simulink library "MidrangeBtc"  (R2022b)
settings: Solver=VariableStepAuto  StartTime=0.0  StopTime=10.0  RelTol=1e-3
undefined symbols (not defined in the file or in its folder): Row
libraries: TuneVar x14, TOP x4, HandyTextFile x2, SetDsm x2, AudioStats x1, FeaturePath x1, RTC x1
settings Model: Creator=st51187  LastModifiedBy=kl13806
settings SolverCC: AlgebraicLoopSolver=TrustRegion
settings DebuggingCC: UnconnectedInputMsg=warning  UnconnectedOutputMsg=warning  UnconnectedLineMsg=warning  SFMachineParentedDataDiag=warning
settings ModelReferenceCC: EnableRefExpFcnMdlSchedulingChecks=on
settings RTWCC: DLArmComputeVersion=19.05

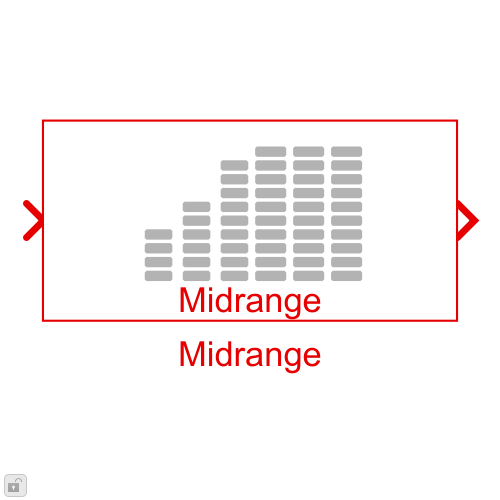
[thumbnail: Simulink's stored preview of the top-level diagram]
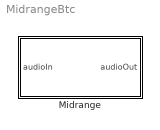
== system MidrangeBtc ==
  Midrange : Subsystem  mask(Blocklib Midrange){FeatureName=Midrange, Config=[]}
      mask prompts: FeatureName "Feature path name:"; Config "MidrangeConfig"
      mask help: The midrange block performs tone controls across midrange frequencies across multiple channels via a 2nd order IIR filter.
      mask init:
      | blkh=gcbh;
      | Config=BTConfig.Assert(blkh,Config);
      | MaskBlockHandle = gcbh;
      | 
      | MidrangeMask.Init(blkh);
      | 
      | % Set boundary conditions
      | rampRateBounds = [5,50000];
      | rampTimeBounds = [1,3000];
      | 
      | BTConfig.InitSetFeatureIfPresent(blkh,'FeatureName');
      | Config.Validate();
      mask Help:
      | The midrange block performs tone controls across midrange frequencies across multiple channels via a 2nd order IIR filter. The midrange content can either be 'boosted' or 'cut' depending on the value of the gain. Different filters can be used for the boost and cut regions, each with its own center frequency and Q value.
      | 
      | MASK PARAMETERS:
      | - Different filter coefficients can be applied for the boost and cut regions (typical center frequency - 775 Hz, Q - 0.9)
      | - The maximum boost/ cut can be specified (typically 20 dB and -20 dB)
      | - The offset and scale values determine the piecewise linear curve that is used to compute the gain (typically 128 and 127 respectively)
      | 
      | RTC CONTROL:
      | Run time control is available to dynamically change the gain to be applied to the midrange content. An index (typically between 0-255) can be provided along with a ramp time and rate (rate gets precedence).
      | RTC_SIM_OBJ.AddREQ( 'MidrangeSet', 0.6, [0005,  <midrange_index>, <ramp_db_per_second>, <ramp_time>]);
      | E.g., RTC_SIM_OBJ.AddREQ( 'MidrangeSet', 0.6, [0005,  50, 0, 50]);
      mask TypeOptions FeatureName: FeaturePath/FeatureName
      mask Callback Config: BTConfig.CallbackHideIfPresent(gcbh,{'FeatureName'});
      mask Display:
      | [path w h] = IconToneMask();
      | 
      | % retrieve the block's pixel size
      | pos = get(gcbh,'position');
      | bw = pos(3) - pos(1);
      | bh = pos(4) - pos(2);
      | 
      | % draw centered icon
      | xAdj = bw/2 - w/2;
      | yAdj = bh/2 - h/2 + 4;
      | for i=1:length(path)
      | 	patch(path(i).x+xAdj, path(i).y+yAdj, path(i).rgb);
      | end
      | 
      | % place feature name text
      | 	text(bw*0.5, 0, ['\n' FeatureName '\n\n'], 'horizontalAlignment', 'center');

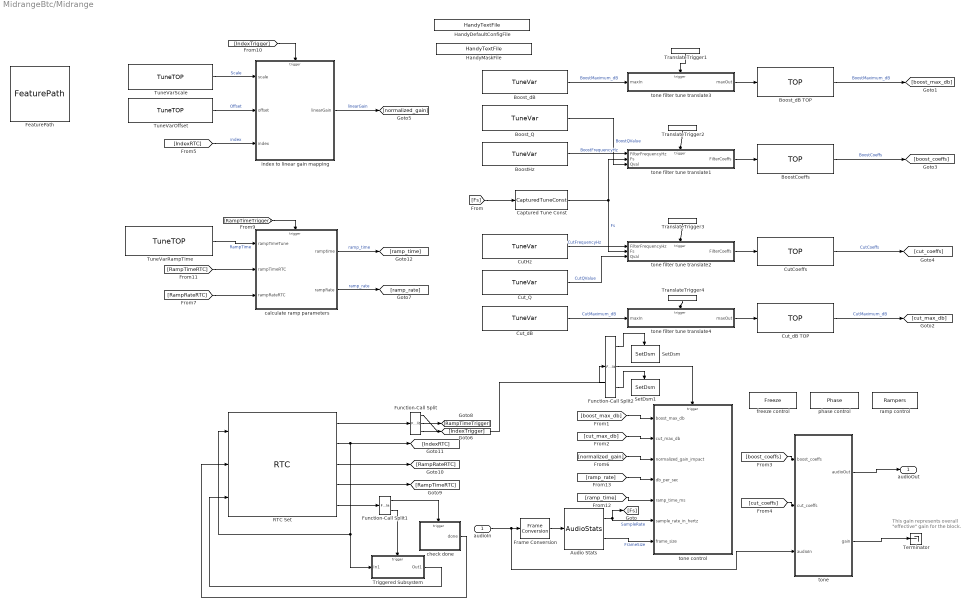
== system MidrangeBtc/Midrange ==
  note: This gain represents overall
      | "effective" gain for the block.
  audioIn : Inport
  Audio Stats : AudioStats/AudioStats  DoSampleRate=on  TypeSampleRate=Inherit: auto  DoCallRate=off  TypeCallRate=Inherit: auto  DoFrameSize=on  TypeFrameSize=Inherit: auto  DoChannelCount=off  TypeChannelCount=Inherit: auto  DoTaskRateFactor=off  TypeTaskRateFactor=Inherit: auto  MacroNameRoot=AUDIO  MacroNameRootEval='AUDIO'  IsMacroNameEval=off  MacroSampleRate=off  MacroCallRate=off  MacroFrameSize=off  MacroChannelCount=off  MacroTaskRateFactor=off  MacroTaskId=off  ValidateSampleRate=off  ValueSampleRate=44100  ValidateCallRate=off  ValueCallRate=[]  ValidateFrameSize=off  ValueFrameSize=32  ValidateChannelCount=off  ValueChannelCount=[]  ValidateTaskRateFactor=off  ValueTaskRateFactor=[]
      settings: SourceProductName=Bose Talaria
  BoostCoeffs : TOP/TOP  TriggerInit=[1775 237 1925 293]  TopName=BoostCoeffs  DataType=single  BankNumber=Config.BankNumber  PreOverlay=false  PostOverlay=false  Role=Automatic
      settings: SourceProductName=Bose Talaria
  BoostHz : TuneVar/TuneVar  Description=Indicates the 'center frequency' of the target frequency band for the 'Boost' filter.  TuneName=BoostFrequencyHz  SpecifyMaxSize=off  VariableDim=1 (Row)  MaxSize=[1 1]  TunabilityNumber=1  MinValue=[]  MaxValue=[]  TriggerInit=[1240 232 1405 278]  MaskValue=Config.DefaultBoostHz
      settings: SourceProductName=Bose Talaria
  Boost_Q : TuneVar/TuneVar  Description=Value represents the width of the frequency band for the 'Boost' filter.  TuneName=BoostQValue  SpecifyMaxSize=off  VariableDim=1 (Row)  MaxSize=[1 1]  TunabilityNumber=1  MinValue=[]  MaxValue=[]  TriggerInit=[1240 160 1405 210]  MaskValue=Config.DefaultBoostq
      settings: SourceProductName=Bose Talaria
  Boost_dB : TuneVar/TuneVar  Description=Indicates the maximum impact in dB for the tone boost. This value must be positive. A negative boost impact would imply a gain cut instead!  TuneName=BoostMaximum_dB  SpecifyMaxSize=off  VariableDim=1 (Row)  MaxSize=[1 1]  TunabilityNumber=1  MinValue=[0]  MaxValue=[]  TriggerInit=[1240 92 1405 138]  MaskValue=Config.DefaultBoostDb
      settings: SourceProductName=Bose Talaria
  Boost_dB TOP : TOP/TOP  TriggerInit=[1775 87 1925 143]  TopName=BoostMaximum_dB  DataType=single  BankNumber=Config.BankNumber  PreOverlay=false  PostOverlay=false  Role=Automatic
      settings: SourceProductName=Bose Talaria
  Captured Tune Const : TuneVar/CapturedTuneConst  TriggerInit=[1305 327 1405 363]  Role=Automatic
      settings: SourceProductName=Bose Talaria
  CutCoeffs : TOP/TOP  TriggerInit=[1775 417 1925 473]  TopName=CutCoeffs  DataType=single  BankNumber=Config.BankNumber  PreOverlay=false  PostOverlay=false  Role=Automatic
      settings: SourceProductName=Bose Talaria
  CutHz : TuneVar/TuneVar  Description=Indicates the 'center frequency' of the target frequency band for the 'Cut' filter.  TuneName=CutFrequencyHz  SpecifyMaxSize=off  VariableDim=1 (Row)  MaxSize=[1 1]  TunabilityNumber=1  MinValue=[]  MaxValue=[]  TriggerInit=[1240 412 1405 458]  MaskValue=Config.DefaultCutHz
      settings: SourceProductName=Bose Talaria
  Cut_Q : TuneVar/TuneVar  Description=Value represents the width of the frequency band for the 'Cut' filter.  TuneName=CutQValue  SpecifyMaxSize=off  VariableDim=1 (Row)  MaxSize=[1 1]  TunabilityNumber=1  MinValue=[0]  MaxValue=[]  TriggerInit=[1240 482 1405 528]  MaskValue=Config.DefaultCutq
      settings: SourceProductName=Bose Talaria
  Cut_dB : TuneVar/TuneVar  Description=Indicates the maximum impact in dB for the tone cut. This value must be positive. A negative cut impact would imply a gain boost instead!  TuneName=CutMaximum_dB  SpecifyMaxSize=off  VariableDim=1 (Row)  MaxSize=[1 1]  TunabilityNumber=1  MinValue=[0]  MaxValue=[]  TriggerInit=[1240 552 1405 598]  MaskValue=Config.DefaultCutDb
      settings: SourceProductName=Bose Talaria
  Cut_dB TOP : TOP/TOP  TriggerInit=[1775 547 1925 603]  TopName=CutMaximum_dB  DataType=single  BankNumber=Config.BankNumber  PreOverlay=false  PostOverlay=false  Role=Automatic
      settings: SourceProductName=Bose Talaria
  FeaturePath : FeaturePath/FeaturePath  FeatureName=Midrange  IsGroup=off  GroupNumber=-1  IsModule=off  TriggerInit=[320 84 435 191]
      settings: SourceProductName=Bose Talaria
  Frame Conversion : FrameConversion  OutFrame=Sample-based
  Function-Call Split : FunctionCallSplit  IconShape=distinctive  NumOutputPorts=3
  Function-Call Split1 : FunctionCallSplit  IconShape=distinctive  NumOutputPorts=2  OutputPortLayout=default
  Function-Call Split2 : FunctionCallSplit  IconShape=distinctive  NumOutputPorts=3  OutputPortLayout=default
  HandyDefaultConfigFile : HandyTextFile/HandyTextFile  TemplateSource=Config  FileSuffix=Init  OpenDialogOnLoad=off  UseThisBlockName=off  AddGrandParentNamePrefix=off  TheDefaultText=|  ShowInLibBrowser=on
      | % $(FILENAME) Setup model parameters for each "Init" callback (e.g. update diagram)
      | sample_rate_in_hertz = 44100;
      | frame_size = 32;
      | sysin_channel_count = 2;
      settings: SourceProductName=Bose Talaria
  HandyMaskFile : HandyTextFile/HandyTextFile  TemplateSource=<dialog fields>  FileSuffix=Mask  OpenDialogOnLoad=off  UseThisBlockName=off  AddGrandParentNamePrefix=off  TheDefaultText=|  ShowInLibBrowser=on
      | % $(FILENAME) Setup model parameters for each "Init" callback (e.g. update diagram)
      | sample_rate_in_hertz = 44100;
      | frame_size = 32;
      | sysin_channel_count = 2;
      settings: SourceProductName=Bose Talaria
  RTC Set : RTC/RTC  REQ_Priority=RTC_Mask.NormalPriority  RequestAtInit=off  EnableRequest=on  REQElemName1=gain_index  REQElemType1=uint32  REQElemWidth1=1  REQElemInitial1=[]  REQElemName2=ramp_db_per_second  REQElemType2=uint32  REQElemWidth2=1  REQElemInitial2=[]  REQElemName3=ramp_milliseconds  REQElemType3=uint32  REQElemWidth3=1  REQElemInitial3=[]  REQElemType4=uint32  REQElemWidth4=1  REQElemInitial4=[]  REQElemType5=uint32  REQElemWidth5=1  REQElemInitial5=[]  REQElemType6=uint32  REQElemWidth6=1  REQElemInitial6=[]  REQElemType7=uint32  REQElemWidth7=1  REQElemInitial7=[]  REQElemType8=uint32  REQElemWidth8=1  REQElemInitial8=[]  REQElemType9=uint32  REQElemWidth9=1  REQElemInitial9=[]  REQElemType10=uint32  REQElemWidth10=1  REQElemInitial10=[]  EnableResponse=on  EnableRSP_StatusIn=off  RSPElemName1=gain_index  RSPElemType1=uint32  RSPElemWidth1=1  RSPElemType2=uint32  RSPElemWidth2=1  RSPElemType3=uint32  RSPElemWidth3=1  RSPElemType4=uint32  RSPElemWidth4=1  RSPElemType5=uint32  RSPElemWidth5=1  RSPElemType6=uint32  RSPElemWidth6=1  RSPElemType7=uint32  RSPElemWidth7=1  RSPElemType8=uint32  RSPElemWidth8=1  RSPElemType9=uint32  RSPElemWidth9=1  RSPElemType10=uint32  RSPElemWidth10=1  EnableNotification=on  EnableNTF_PrepTrig=off  NTFElemName1=gain_index  NTFElemType1=uint32  NTFElemWidth1=1  NTFElemType2=uint32  NTFElemWidth2=1  NTFElemType3=uint32  NTFElemWidth3=1  NTFElemType4=uint32  NTFElemWidth4=1  NTFElemType5=uint32  NTFElemWidth5=1  NTFElemType6=uint32  NTFElemWidth6=1  NTFElemType7=uint32  NTFElemWidth7=1  NTFElemType8=uint32  NTFElemWidth8=1  NTFElemType9=uint32  NTFElemWidth9=1  NTFElemType10=uint32  NTFElemWidth10=1  MaskMessageName=Set
      settings: SourceProductName=Bose Talaria
  SetDsm : SetDsm/SetDsm  DataStoreName=Freeze  Value=uint32(1)
      settings: SourceProductName=Bose Talaria
  SetDsm1 : SetDsm/SetDsm  DataStoreName=Freeze  Value=uint32(0)
      settings: SourceProductName=Bose Talaria
  Terminator : Terminator
  TranslateTrigger1 : TuneVar/TranslateTrigger  TriggerInit=[1608 50 1662 60]
      settings: SourceProductName=Bose Talaria
  TranslateTrigger2 : TuneVar/TranslateTrigger  TriggerInit=[1603 200 1657 210]
      settings: SourceProductName=Bose Talaria
  TranslateTrigger3 : TuneVar/TranslateTrigger  TriggerInit=[1603 380 1657 390]
      settings: SourceProductName=Bose Talaria
  TranslateTrigger4 : TuneVar/TranslateTrigger  TriggerInit=[1603 530 1657 540]
      settings: SourceProductName=Bose Talaria
  Triggered Subsystem : Subsystem  TreatAsAtomicUnit=on
  TuneVarOffset : TuneVar/TuneTOP  Description=Offset represents the midpoint of the index range, which separates the 'boost' indices from the 'cut' indices.  TriggerInit=[550 147 715 193]  TopName=Offset  TuneName=Offset  DataType=single  TunabilityNumber=1  MinValue=[]  MaxValue=[]  BankNumber=0  PreOverlay=false  PostOverlay=false  UseSameName=on  MaskValue=Config.DefaultDefaultOffset
      settings: SourceProductName=Bose Talaria
  TuneVarRampTime : TuneVar/TuneTOP  Description=This is the default ramp time that will be used if the RTC message has a '0' for both ramp time and ramp rate.  TriggerInit=[545 397 715 453]  TopName=RampTime  TuneName=RampTime  DataType=single  TunabilityNumber=1  MinValue=1  MaxValue=100000  BankNumber=0  PreOverlay=false  PostOverlay=false  UseSameName=on  MaskValue=30
      settings: SourceProductName=Bose Talaria
  TuneVarScale : TuneVar/TuneTOP  Description=Scale is used to normalize the linear gain to a value between +/- 1. The range (0,1] represents a boost while the range [-1,0) represents a cut. We use the number of available indices in each range (mapped to gain values between [-1,1]) as the denominator for normalization, i.e. as the 'Scale'.  TriggerInit=[550 81 715 129]  TopName=Scale  TuneName=Scale  DataType=single  TunabilityNumber=1  MinValue=[]  MaxValue=[]  BankNumber=0  PreOverlay=false  PostOverlay=false  UseSameName=on  MaskValue=Config.DefaultDefaultScale
      settings: SourceProductName=Bose Talaria
  calculate ramp parameters : MATLAB Function  TreatAsAtomicUnit=on
  check done : MATLAB Function  TreatAsAtomicUnit=on
  freeze control : DataStoreMemory  DataStoreName=Freeze  ShowAdditionalParam=off  OutDataTypeStr=uint32
  index to linear gain mapping : MATLAB Function  TreatAsAtomicUnit=on
  phase control : DataStoreMemory  DataStoreName=Phase  InitialValue=1  ShowAdditionalParam=off  OutDataTypeStr=uint32
  ramp control : DataStoreMemory  DataStoreName=Rampers  InitialValue=Config.DlgRamperInit  ShowAdditionalParam=off  OutDataTypeStr=Bus: rgain_bus
  tone : MATLAB Function  TreatAsAtomicUnit=on
  tone control : MATLAB Function  TreatAsAtomicUnit=on
  tone filter tune translate1 : MATLAB Function  TreatAsAtomicUnit=on
  tone filter tune translate2 : MATLAB Function  TreatAsAtomicUnit=on
  tone filter tune translate3 : MATLAB Function  TreatAsAtomicUnit=on
  tone filter tune translate4 : MATLAB Function  TreatAsAtomicUnit=on
  audioOut : Outport  VectorParamsAs1DForOutWhenUnconnected=off
  wires:
  CutHz/1 -> tone filter tune translate2/1(FilterFrequencyHz)  "CutFrequencyHz"
  TuneVarScale/1 -> index to linear gain mapping/1(scale)  "Scale"
  Boost_Q/1 -> tone filter tune translate1/3(Qval)  "BoostQValue"
  Cut_dB TOP/1 -> [cut_max_db]  "CutMaximum_dB"
  Audio Stats/1 -> tone control/6(sample_rate_in_hertz), [Fs]  "SampleRate"
  calculate ramp parameters/2(rampRate) -> [ramp_rate]  "ramp_rate"
  [boost_max_db] -> tone control/1(boost_max_db)
  [boost_coeffs] -> tone/1(boost_coeffs)
  tone filter tune translate3/1(maxOut) -> Boost_dB TOP/1
  BoostCoeffs/1 -> [boost_coeffs]  "BoostCoeffs"
  Boost_dB/1 -> tone filter tune translate3/1(maxIn)  "BoostMaximum_dB"
  Frame Conversion/1 -> Audio Stats/1
  Cut_dB/1 -> tone filter tune translate4/1(maxIn)  "CutMaximum_dB"
  RTC Set/1 -> Function-Call Split/1
  audioIn/1 -> tone/3(audioIn), Frame Conversion/1
  tone filter tune translate1/1(FilterCoeffs) -> BoostCoeffs/1
  CutCoeffs/1 -> [cut_coeffs]  "CutCoeffs"
  Captured Tune Const/1 -> tone filter tune translate1/2(Fs), tone filter tune translate2/2(Fs)  "Fs"
  tone filter tune translate4/1(maxOut) -> Cut_dB TOP/1
  check done/1(done) -> RTC Set/2
  RTC Set/2 -> Triggered Subsystem/1(In1), RTC Set/1, [IndexRTC]
  TranslateTrigger3/1 -> tone filter tune translate2/Trigger
  Function-Call Split/1 -> [IndexTrigger]
  TranslateTrigger2/1 -> tone filter tune translate1/Trigger
  Audio Stats/2 -> tone control/7(frame_size)  "FrameSize"
  BoostHz/1 -> tone filter tune translate1/1(FilterFrequencyHz)  "BoostFrequencyHz"
  [RampRateRTC] -> calculate ramp parameters/3(rampRateRTC)
  TranslateTrigger4/1 -> tone filter tune translate4/Trigger
  TuneVarOffset/1 -> index to linear gain mapping/2(offset)  "Offset"
  Cut_Q/1 -> tone filter tune translate2/3(Qval)  "CutQValue"
  [IndexRTC] -> index to linear gain mapping/3(index)  "index"
  TranslateTrigger1/1 -> tone filter tune translate3/Trigger
  [RampTimeTrigger] -> calculate ramp parameters/Trigger
  TuneVarRampTime/1 -> calculate ramp parameters/1(rampTimeTune)  "RampTime"
  [RampTimeRTC] -> calculate ramp parameters/2(rampTimeRTC)
  [IndexTrigger] -> index to linear gain mapping/Trigger
  calculate ramp parameters/1(ramptime) -> [ramp_time]  "ramp_time"
  tone/1(audioOut) -> audioOut/1
  tone/2(gain) -> Terminator/1
  Function-Call Split/3 -> Function-Call Split2/1
  RTC Set/3 -> [RampRateRTC]
  RTC Set/4 -> [RampTimeRTC]
  tone filter tune translate2/1(FilterCoeffs) -> CutCoeffs/1
  [ramp_time] -> tone control/5(ramp_time_ms)
  index to linear gain mapping/1(linearGain) -> [normalized_gain]  "linearGain"
  [Fs] -> Captured Tune Const/1
  [cut_coeffs] -> tone/2(cut_coeffs)
  Function-Call Split/2 -> [RampTimeTrigger]
  [normalized_gain] -> tone control/3(normalized_gain_impact)
  [cut_max_db] -> tone control/2(cut_max_db)
  Boost_dB TOP/1 -> [boost_max_db]  "BoostMaximum_dB"
  [ramp_rate] -> tone control/4(db_per_sec)
  RTC Set/5 -> Function-Call Split1/1
  Function-Call Split1/1 -> check done/Trigger
  Function-Call Split1/2 -> Triggered Subsystem/Trigger
  Triggered Subsystem/1(Out1) -> RTC Set/3
  Function-Call Split2/2 -> tone control/Trigger
  Function-Call Split2/3 -> SetDsm1/Trigger
  Function-Call Split2/1 -> SetDsm/Trigger

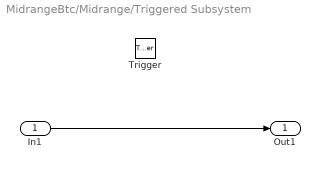
== system MidrangeBtc/Midrange/Triggered Subsystem ==
  In1 : Inport
  Trigger : TriggerPort  TriggerType=function-call  VariantControl=Variant
  Out1 : Outport
  wires:
  In1/1 -> Out1/1

== matlab function MidrangeBtc/Midrange/tone control ==
  data: boost_max_db input; cut_max_db input; Rampers data_store_memory; normalized_gain_impact input; db_per_sec input; ramp_time_ms input; sample_rate_in_hertz input; frame_size input; Phase data_store_memory
  events: trigger input FUNCTION_CALL_EVENT
function control(...
    boost_max_db, cut_max_db, ...
    normalized_gain_impact, db_per_sec, ramp_time_ms, sample_rate_in_hertz, frame_size)

% See Controlsummary at the end;

global Phase;
global Rampers;

rgain_SILENT_GAIN = RgainBusUtil.GetSilentGainLinear();

% Step 1: FREEZE the gain ramper so that we can perform calculations based
% on the current gain value. (This step now performed on canvas)

% Step 2a: IMPACT-TARGET Translate the normalized gain into a dB impact
% based on the maximum boost or cut values.
% ("-1" = maximum cut, "1" = maximum boost.)
[targetIsBoost,targetImpact_db,targetEffectiveGain,...
    actualTargetGainLinear] = ...
    tone_control_split1(normalized_gain_impact,boost_max_db,cut_max_db);

% Step 2b: IMPACT-CURRENT Fetch the current gain from the previously
% active ramper.
currentPhase = Phase;
currentGain = Rampers(currentPhase).currentGain;
currentIsBoost = (currentGain >= 1);
currentImpact_db = db20(currentGain);

% Setup processing to continue on seamlessly while we work here
Rampers(1).currentGain = currentGain;
Phase = uint32(1); % reset phase to 1
% Now that we have both current and target impacts, find the difference
db_diff = abs(currentImpact_db - targetImpact_db);

% Step 3a: TIME- If a slope in dB/second is provided, ignore the ramp time
% and instead calculate a new ramp time that matches the slope.
if (db_per_sec)
    ramp_ms = db_diff / single(db_per_sec) * 1000;
else
    ramp_ms = single(ramp_time_ms);
end

% Step 3b: TIME- QUANTIZE the desired ramp time to our FrameSize. 
quantum_ms = 1000 * frame_size / sample_rate_in_hertz;
numFrames = ramp_ms / quantum_ms;
numFrames = max (1, ceil(numFrames));

% Step 4a: PHASES- Determine whether ramping from current gain to target
% gain requires a unity crossing in linear gain. 
isTwoPhase = (currentIsBoost ~= targetIsBoost) && ...
    (currentGain ~= 1) && ... % cannot cross if you're already there
    (targetImpact_db ~= 1);  % no crossing needed when impact already nothing
% Setup a structure to hold information about what the rampers should do
twoSingles = {single(0) single(0)};
phaseConfig = struct('frames',twoSingles,'target_linear',twoSingles,'current_linear',twoSingles);
phaseConfig = tone_control_split2(numFrames,currentImpact_db,...
    db_diff,currentGain,currentIsBoost,rgain_SILENT_GAIN,targetIsBoost,...
    targetEffectiveGain,isTwoPhase,phaseConfig);

% Step 4b: PHASES- Setup rampers for both phases
for currentPhase=1:2
    % In order to have the desired ramp time, the slope must vary dependent
    % on the gain difference between target and current value.
    % Ramper's coefficient is therefore calculated as follows:

    if (phaseConfig(currentPhase).frames)
        ramp_ms = quantum_ms * phaseConfig(currentPhase).frames;
        factor = log(phaseConfig(currentPhase).target_linear / phaseConfig(currentPhase).current_linear);
        RampCoef = exp(factor / (sample_rate_in_hertz * ramp_ms / 1000));
    else
        RampCoef = single(1);
    end
    
    % Output control signals
    Rampers(currentPhase).frameCount  = int32(phaseConfig(currentPhase).frames);
    Rampers(currentPhase).rampCoeff   = single(RampCoef);
    Rampers(currentPhase).targetGain  = actualTargetGainLinear; % phase 1 value ignored.
    Rampers(currentPhase).currentGain = single(phaseConfig(currentPhase).current_linear);
end

% unfreeze the gain (This step now performed on canvas)

end

% Nudge the gain values a bit if they are sitting right at one (aka unity).
% When a control set goes live, ensure that the current gain will move.
% If current gain is one, replace with a value very close to one. What we
% really want is a value which is on the edge of perception - not too small
% or large. If the value is too small, we'll waste some of our ramp time
% in perceived silence. If the value is too large, the audio will lurch
% into perceptability at the start of the ramp. Remember that normally we
% worry about gains of 0 -- this checks instead against 1 because filter
% gain is effective gain minuus 1.
function adjustedLinearGain = NudgeUnity(linearGain,isPositive,silentGain)
if (isPositive)
    adjustedLinearGain = max(linearGain, 1 + silentGain);
else
    adjustedLinearGain = min(linearGain, 1 - silentGain);
end
end % NudgeUnity end

function [targetIsBoost,targetImpact_db,targetEffectiveGain,...
    actualTargetGainLinear] = ...
    tone_control_split1(normalized_gain_impact,boost_max_db,cut_max_db)
targetIsBoost = (normalized_gain_impact >= 0);
if (targetIsBoost)
    targetImpact_db = normalized_gain_impact * boost_max_db;
    targetEffectiveGain = undb20(targetImpact_db); % 1 or greater
else
    targetImpact_db = normalized_gain_impact * cut_max_db;
    targetEffectiveGain = undb20(targetImpact_db); % less than 1
end
% remember the actual target because we will nudge this value away from one
% during the ramper calculations. This actual target value is used below as
% the target in the ramper data itself.
actualTargetGainLinear = targetEffectiveGain;

end %tone_control_split1


function phaseConfig = tone_control_split2(numFrames,currentImpact_db,...
    db_diff,currentGain,currentIsBoost,rgain_SILENT_GAIN,targetIsBoost,...
    targetEffectiveGain,isTwoPhase,phaseConfig)

if (isTwoPhase)
    % Both boost and cut phases will be required to get where we are going.
    % Make sure we have at least two frames to work with:
    numFrames = max (2, round(numFrames));
    
    % Divide up our ramp time into pieces for each phase to use
    phase1Frames = ceil(numFrames * abs(currentImpact_db) / db_diff);
    phase2Frames = numFrames - phase1Frames;
    
    % Make sure phase 2 has at least 1 frame to work with
    phase2Frames = max(1, phase2Frames);
    
    % Setup Phase 1 ramper that takes us to zero impact (i.e. unity gain)
    phaseConfig(1).current_linear   = currentGain;  % we know this is not 1
    phaseConfig(1).target_linear    = NudgeUnity(1,currentIsBoost,rgain_SILENT_GAIN);
    phaseConfig(1).frames           = phase1Frames;
    
    % Setup Phase 2 ramper that delivers us to target impact
    phaseConfig(2).current_linear   = NudgeUnity(1,targetIsBoost,rgain_SILENT_GAIN); % start quiet
    phaseConfig(2).target_linear    = targetEffectiveGain;   % we know this is not 0
    phaseConfig(2).frames           = phase2Frames;
else
    % Only one phase is needed to accomplish our goal. We are are the
    % target side of unity... but we must determine which side that is
    if (currentGain == 1)
        % One is in-between sides: use the target to determine the side
        isBoost = targetIsBoost;
    else
        % Current gain is already on one side of unity so use that
        isBoost = currentIsBoost;
    end
    phaseConfig(1).current_linear   = NudgeUnity(currentGain,isBoost,rgain_SILENT_GAIN);
    phaseConfig(1).target_linear    = NudgeUnity(targetEffectiveGain,isBoost,rgain_SILENT_GAIN);
    phaseConfig(1).frames           = numFrames;
    
    % Setup Phase 2 ramper to sit at the target gain
    phaseConfig(2).current_linear   = NudgeUnity(targetEffectiveGain,isBoost,rgain_SILENT_GAIN);
    phaseConfig(2).target_linear    = NudgeUnity(targetEffectiveGain,isBoost,rgain_SILENT_GAIN);
    phaseConfig(2).frames           = single(0);
end

end %tone_control_split2

% This routine sets up the control data that directs the operation of
% the signal processing logic. The high level design of the tone block
% involves filtering out frequency range of the signal and then mixing it
% back in. This results in a boost or a cut to the filtered frequencies. As
% such, the gain of the filtered signal equals the overall tone block's
% effective gain minus 1 for the unfiltered signal.
%
% FilterGain = EffectiveGain - 1
%                             _
%                            / \   EffectiveGain
%   >-------+-------------->| + |------------------>
%           |                \ /
%           v                 |
%      +----+---+             ^
%      |        |            / \
%      | Filter |           /   \ FilterGain
%      |        |          /gain \
%      +----+---+          +-----+
%           |                 ^
%           |                 |
%           +-----------------+
%
% Another issue of note is that crossing over from boost to cut or vice
% versa involves numerically crossing 0 in terms of the filter gain (or
% crossing 1 in terms of effective gain). When the intended impact is 0 the
% filter gain is 0... so no impact to signal because the filtered signal is
% attenuated to 0. Since filter gain changes exponentially so as to be
% linear in dB space, it is impossible to cross past 0 (from boosting to
% cutting for instance) via multiplication alone. To combat this challenge,
% this block enlists two rampers. When a single gain change involves
% crossing over the boost/cut boundary, the first ramper takes gain up yo
% the boundary and then the second ramper is set up to continue the journey
% on the other side of the boundary to ultimately reach the target impact
% gain.
%
% Inputs:
%   boost_max_db, cut_max_db: indicates maximum impact of tone impact in dB
%        which must be positive. A negative cut dB would imply a boost!
%   normalized_gain_impact : Target impact of the tone filter that must be
%        between -1 and 1. A value of "0" implies no effect, 1 and -1 are
%        maximum boost and cut respectively.
% Control Data:
%   FreezePhase(1) freezes the processing during this control operation
%   FreezePhase(2) indicates the current phase- always reset here to 1. The
%        phase indicates which of the two rampers is active. Once the first
%        ramper finishes, the second takes over (potentially to do
%        nothing if the adjustment did not require a boost/cut crossing)
%   Rampers(1) is the first phase ramper. Boost vs. cut is determined by
%        the sign of the linear current gain.
%   Rampers(2) is the second phase ramper. Boost vs. cut is determined by
%        the sign of the linear current gain.
%   *Note that the gain present in the rampers is the EFFECTIVE gain (aka
%   filter gain plus one).

% Step 4b: PHASES- Setup rampers for both phases
    % In order to have the desired ramp time, the slope must vary dependent
    % on the gain difference between target and current value.
    % Ramper's coefficient is therefore calculated as follows:
    %
    %   TargetGain = CurrentGain *( RampCoef ^ (Fs*RampTime_ms/1000) )
    %
    % therefore...
    %
    %                     log(TargetGain/CurrentGain)
    %   log(RampCoef) = ------------------------------
    %                        Fs*(RampTime_ms/1000)
    %

== matlab function MidrangeBtc/Midrange/tone filter tune translate1 ==
  data: FilterFrequencyHz input; Fs input; Qval input; FilterCoeffs output
  events: trigger input FUNCTION_CALL_EVENT
function FilterCoeffs  = fcn(FilterFrequencyHz, Fs, Qval)
%#codegen
% Compute the discrete frequency
omega = 2 * pi * FilterFrequencyHz.Value / Fs;
Q = Qval.Value;

% Equations for computing filter coefficients of a bandpass filter
% Compute the denominator coeffs
A1 = (-4 * Q * cos(omega)) / (2 * Q + sin(omega));
A2 = (2 * Q - sin(omega)) / (2 * Q + sin(omega));
% Compute the numerator coeffs
B0 = sin(omega)/ (2 * Q + sin(omega));
B1 = 0;
B2 = -B0;
% Concatenate to obtain the final coeffs
FilterCoeffs = single([A1 A2 B0 B1 B2]);

== matlab function MidrangeBtc/Midrange/tone filter tune translate3 ==
  data: maxOut output; maxIn input
  events: trigger input FUNCTION_CALL_EVENT
function maxOut  = fcn( ...
    maxIn) ... % inputs % parameters
%#codegen

% Just make sure the maximum is a positive dB value
maxOut = single(abs(maxIn.Value));

== matlab function MidrangeBtc/Midrange/tone filter tune translate4 ==
  data: maxOut output; maxIn input
  events: trigger input FUNCTION_CALL_EVENT
function maxOut  = fcn( ...
    maxIn) ... % inputs % parameters
%#codegen

% Just make sure the maximum is a positive dB value
maxOut = single(abs(maxIn.Value));

== matlab function MidrangeBtc/Midrange/tone filter tune translate2 ==
  data: FilterFrequencyHz input; Fs input; Qval input; FilterCoeffs output
  events: trigger input FUNCTION_CALL_EVENT
function FilterCoeffs  = fcn(FilterFrequencyHz, Fs, Qval)
%#codegen
% Compute the discrete frequency
omega = 2 * pi * FilterFrequencyHz.Value / Fs;
Q = Qval.Value;

% Equations for computing filter coefficients of a bandpass filter
% Compute the denominator coeffs
A1 = (-4 * Q * cos(omega)) / (2 * Q + sin(omega));
A2 = (2 * Q - sin(omega)) / (2 * Q + sin(omega));
% Compute the numerator coeffs
B0 = sin(omega)/ (2 * Q + sin(omega));
B1 = 0;
B2 = -B0;
% Concatenate to obtain the final coeffs
FilterCoeffs = single([A1 A2 B0 B1 B2]);

== matlab function MidrangeBtc/Midrange/check done ==
  data: done output; Rampers data_store_memory
  events: trigger input FUNCTION_CALL_EVENT
function done  = fcn
%#codegen

global Rampers;

% Checking whether the frameCounts are exactly equal to 0 was leading to
% unpredictable behavior. Therefore, we now check whether or not the 
% frameCounts are less-than/equal-to 0.
% See SAMPLERATE-1196 & SAMPLERATE-1205 for more details. 
done = (Rampers(1).frameCount <= 0) && (Rampers(2).frameCount <= 0);

== matlab function MidrangeBtc/Midrange/index to linear gain mapping ==
  data: linearGain output; scale input; offset input; index input
  events: trigger input FUNCTION_CALL_EVENT
function linearGain = compute_gain(scale,offset,index)
%#codegen

% The midrange curve is configured as a piecewise linear plot, with
% configurable values of the maximum boost ('maxB') and maximum cut ('maxC')
% in dB. 
%    dB ^
%       |
% maxB  ----------/
%       |        /
%       |       /
%  0    ------|---|----> index
%       |   /128  255
%       |  /
% maxC  --/
%       |
% Hence, for any given index, the gain is calculated as a value in 
% between 0 and 1 for boost and 0 and -1 for cut. This will later be
% multiplied with the maxB or maxC to get the actual gain value. 
% (y - y1) / (x - x1) = (y1 - y2) / (x1 - x2)
% (y - 0) / (x - 128) = (0 - 1) / (128 - 255)
%                   y = (x - 128)/127
% 'offset' represents the center point between boost and cut (i.e. 128) and
% 'scale' represents how many intervals are available for boost/cut (i.e. 127)

% Apply the tuning calibration
floatIndex = single(index);
linearGain = single((floatIndex - offset) / scale);

% Ensure the result is between -1 and 1
linearGain = min(linearGain, 1);
linearGain = max(linearGain, -1);

== matlab function MidrangeBtc/Midrange/calculate ramp parameters ==
  data: ramptime output; rampTimeTune input; rampTimeRTC input; rampRateRTC input; rampRate output; rampRateBounds parameter; rampTimeBounds parameter
  events: trigger input FUNCTION_CALL_EVENT
function [ramptime, rampRate]  = ramp_parameters(...
    rampTimeTune, rampTimeRTC, rampRateRTC,... % inputs
    rampRateBounds, rampTimeBounds) % parameters
%#codegen
    % Ramp time mentioned in the RTC message gets priority over the tune
    % variable. Boundary conditions are also included based on BDSP values.
    
    ramptime = single(rampTimeTune);
    rampRate = single(0);
    
    if (rampRateRTC)
        rampRate = single(rampRateRTC);
        rampRate = max(rampRateBounds(1), rampRate);
        rampRate = min(rampRateBounds(2), rampRate);
    end
    if (rampTimeRTC)
        ramptime = single(rampTimeRTC);
    end
    ramptime = max(rampTimeBounds(1), ramptime);
    ramptime = min(rampTimeBounds(2), ramptime);
end

== matlab function MidrangeBtc/Midrange/tone ==
  data: audioOut output; boost_coeffs input; cut_coeffs input; audioIn input; Rampers data_store_memory; gain output; Freeze data_store_memory; Phase data_store_memory
function [audioOut,gain] ...
    = toneProcess(boost_coeffs, cut_coeffs, audioIn)...    % inputs % parameters
  
%#codegen

% Data Store objects (registered in "Edit Data" dialog
global Rampers;
global Freeze;
global Phase;

% Keep memory for the filter persistent from frame to frame
persistent toneFilterStates;

% figure out the frame size and channel count
[frame_size, channel_count] = size(audioIn);

if (isempty(toneFilterStates))
    toneFilterStates = zeros(2,channel_count,'single');
end

% set the size and datatype of the output buffer
audioOut = coder.nullcopy(audioIn);

ramper = Phase;
ramperCount = numel(Rampers);

if (Freeze == false)
    if (Rampers(ramper).frameCount == 0)
        % The current ramper is finished. Is there another one?
        if (ramper < ramperCount && Rampers(ramper+1).frameCount > 0)
            % Yes - move on to the next phase
            ramper = ramper + 1;
            Phase = ramper;
            k = Rampers(ramper).rampCoeff;
            gain = Rampers(ramper).currentGain;
            Rampers(ramper).frameCount = Rampers(ramper).frameCount - 1;
        else
            %  Stop ramping and SNAP to the target
            k = single(1);
            gain = Rampers(ramper).targetGain;
            % Update completion flag
         end
    else
        % The ramp is *NOT* frozen or done: gain is moving
        k = Rampers(ramper).rampCoeff;
        gain = Rampers(ramper).currentGain;
        Rampers(ramper).frameCount = Rampers(ramper).frameCount - 1;
    end
else
    % Frozen. Stay at current gain
    k = single(1);
    gain = Rampers(ramper).currentGain;
end

% Apply the tone filter
if (gain < 1)
    % Cut
    aCoeffs = cut_coeffs(1:2);
    bCoeffs = cut_coeffs(3:5);    
else
    % Boost
    aCoeffs = boost_coeffs(1:2);
    bCoeffs = boost_coeffs(3:5);
end

% [filtered,toneFilterStates] = filter(bCoeffs, aCoeffs, audioIn, toneFilterStates);

% Loop through samples, adjusting gain and applying to channels
for n=1:frame_size
    % Update the gain and then subtract one before applying it to the
    % filtered signal. Disregarding phase shifting 
    gain = gain * k;
    filterGain = gain - 1;
    % Loop through channels adding in gain-adjusted filtered samples
    for chanIdx = 1:channel_count
        
        filterOut = (bCoeffs(1) * audioIn(n,chanIdx)) + toneFilterStates(1,chanIdx);
        toneFilterStates(1,chanIdx) = toneFilterStates(2,chanIdx) - aCoeffs(1) * filterOut;
        toneFilterStates(2,chanIdx) = bCoeffs(3) * audioIn(n,chanIdx) - (aCoeffs(2) * filterOut);
        
        audioOut(n,chanIdx) = audioIn(n,chanIdx) + (filterOut * filterGain);
    end
end

Rampers(ramper).currentGain = gain;
